simulink model "ZEH_PV_grid"  (R2020a)
settings: Solver=VariableStepAuto  StartTime=0.0  StopTime=24*60*60  RelTol=1e-3
InitFcn:
  | SENSE2_dat
values from neighbouring files (symbols this model uses):
  apv = [72 76 288 252 0 0 40 360 460 168 84]  *1E2    [ZEH_dat_summer.m]    (also in ZEH_dat_winter.m)
  cab = [0.206 0.29 0.36 285 335 ... (first row only)    [ZEH_dat_summer.m]    (also in ZEH_dat_winter.m)
  cons = [0.64,0.60,0.58,0.56,0.56,0.58,0.64,0.76,0.87,0.95,0.99,1.00,0.99,1.00,1.00,0.97,0.96,0.96,0.93,0.92,0.92,0.93,0.87,0.72]    [ZEH_dat_summer.m]    (also in ZEH_dat_winter.m = [0.67,0.63,0.60,0.59,0.59,0.60,0.74,0.86,0.85,0.96,0.96,0.95)
  inic = 0.00095    [ZEH_dat_summer.m]    (also in ZEH_dat_winter.m)
  irr = [0,0,0,0,0,0,0,0,0,0,0,0,0,0,0,0,0,0,0,0,0,0,0,0,0,0,0,0,0,0,0,0,0,0,0,0,0,0,0,0,0,0,0,0,0,0,0,0,0,0,0,0,0,0,0,0,0,0,0,0,0,0,0,0,0,0,0,0,0,0,0,0,0,0,0,0,0,0,0,0,0,0,0,0,0,0,0,0,0,0,0,0,0,0,0,0,0,0,0,0,0,0,0,0,0,0,0,0,0,0,0,0,0,0,0,0,0,0,0,0,0,0,0,0,0,0,0,0,0,0,0,0,0,0,0,0,0,0,0,0,0,0,0,0,0,0,0,0,0,0,0,0,0,0,0,0,0,0,0,0,0,0,0,0,0,0,0,0,0,0,0,0,0,0,0,0,0,0,0,0,0,0,0,0,0,0,0,0,0,0,0,0,0,0,0,0,0,0,0,0 ...(+12851 chars)    [ZEH_dat_summer.m]    (also in ZEH_dat_winter.m = zeros(1,length(irr)))
  lp = 0.002    [ZEH_dat_summer.m]    (also in ZEH_dat_winter.m)
  SL = [7.57 8.06 30.73 53.01 133.26 219.22 4.00 37.53 48.38 17.80 9.04]*1E-3    [ZEH_dat_summer.m]    (also in ZEH_dat_winter.m)
  time = [1,1.01666666666667,1.03333333333333,1.05000000000000,1.06666666666667,1.08333333333333,1.10000000000000,1.11666666666667,1.13333333333333,1.15000000000000,1.16666666666667,1.18333333333333,1.20000000000000,1.21666666666667,1.23333333333333,1.25000000000000,1.26666666666667,1.28333333333333,1.30000000000000,1.31666666666667,1.33333333333333,1.35000000000000,1.36666666666667,1.38333333333333,1.4000 ...(+22733 chars)    [ZEH_dat_summer.m]    (also in ZEH_dat_winter.m)
  to = 0.1    [ZEH_dat_summer.m]    (also in ZEH_dat_winter.m)
undefined symbols (not defined in the file or in its folder): A, B, C, D1, Dd, Delta, j
libraries: powerlib x166, simulink_extras x12, powerlib_meascontrol x11, simulink x2, factslib x2
(part 4 of 5)

== system ZEH_PV_grid/L5/Avoid division by zero ==
  I : Inport
  Complex to Magnitude-Angle : ComplexToMagnitudeAngle
  Magnitude-Angle to Complex : MagnitudeAngleToComplex
  Saturation1 : Saturate  UpperLimit=inf  LowerLimit=1e-6
  O : Outport  VectorParamsAs1DForOutWhenUnconnected=off
  wires:
  I/1 -> Complex to Magnitude-Angle/1
  Saturation1/1 -> Magnitude-Angle to Complex/1
  Complex to Magnitude-Angle/1 -> Saturation1/1
  Magnitude-Angle to Complex/1 -> O/1
  Complex to Magnitude-Angle/2 -> Magnitude-Angle to Complex/2

== system ZEH_PV_grid/L5/Break Alg. Loop 1 ==
  In : Inport
  Complex to Real-Imag : ComplexToRealImag
  Real-Imag to Complex : RealImagToComplex
  imag : Subsystem  mask(Transfer Function with Initial Outputs){N=[1], D=[to  1], Y0=0, U0=0}
      mask prompts: N "Numerator:"; D "Denominator:"; Y0 "Initial output:"; U0 "Initial input:"
      mask help: Vector expressions for numerator, and denominator. Coefficients are in descending powers of s.
      mask init:
      | [A,B,C,Dd]=tf2ss(N,D);if (isempty(Y0));[m,n]=size(A);X0=zeros(1,m); end; if (isempty(U0));[m,p]=size(B);U0=zeros(1,p);end;X0=getxo(A,B,C,Dd,U0,Y0,0);
      mask Help: Specify the initial output for the transfer function.  An optimization routine attempts to determine the appropriate initial states so that the specified initial output is achieved.  For more details, see the m-file getxo.m
      mask Display: dpoly(N,D,'s')
  real : Subsystem  mask(Transfer Function with Initial Outputs){N=[1], D=[to 1], Y0=0, U0=0}
      mask prompts: N "Numerator:"; D "Denominator:"; Y0 "Initial output:"; U0 "Initial input:"
      mask help: Vector expressions for numerator, and denominator. Coefficients are in descending powers of s.
      mask init:
      | [A,B,C,Dd]=tf2ss(N,D);if (isempty(Y0));[m,n]=size(A);X0=zeros(1,m); end; if (isempty(U0));[m,p]=size(B);U0=zeros(1,p);end;X0=getxo(A,B,C,Dd,U0,Y0,0);
      mask Help: Specify the initial output for the transfer function.  An optimization routine attempts to determine the appropriate initial states so that the specified initial output is achieved.  For more details, see the m-file getxo.m
      mask Display: dpoly(N,D,'s')
  Out : Outport  VectorParamsAs1DForOutWhenUnconnected=off
  wires:
  Complex to Real-Imag/1 -> real/1(In1)
  Complex to Real-Imag/2 -> imag/1(In1)
  In/1 -> Complex to Real-Imag/1
  Real-Imag to Complex/1 -> Out/1
  real/1(Out1) -> Real-Imag to Complex/1
  imag/1(Out1) -> Real-Imag to Complex/2

== system ZEH_PV_grid/L5/Load ==
  1 : Constant
  Add : Sum
  Clock : Clock
  Constant : Constant
  Constant1 : Constant  Value=15/24
  Divide : Product  Inputs=*/
  Manual Switch : ManualSwitch
  Mux : Mux  Inputs=2
  P nom : Constant  Value=-nomPower*1e6
  Power consumption : Lookup_n-D  NumberOfTableDimensions=1  BreakpointsForDimension1=[1:timestep/60:24]  BeginIndexSearchUsingPreviousIndexResult=on  Table=datas  InternalRulePriority=Speed  RndMeth=Simplest  InputSameDT=on
  Power factor : Constant  Value=PF^2
  Product : Product
  Product1 : Product
  Scope : Scope
  Second-->Hour : Gain  Gain=1/(60*60)
  Sqrt : Sqrt  SaturateOnIntegerOverflow=on
  Sum : Sum  Inputs=-+
  PQ : Outport  VectorParamsAs1DForOutWhenUnconnected=off
  wires:
  Constant/1 -> Add/2
  1/1 -> Sum/1, Divide/1
  Second-->Hour/1 -> Add/1
  Sum/1 -> Sqrt/1
  Power factor/1 -> Divide/2
  Add/1 -> Power consumption/1
  P nom/1 -> Product/2
  Clock/1 -> Second-->Hour/1
  Sqrt/1 -> Product1/2
  Product/1 -> Product1/1, Mux/1
  Divide/1 -> Sum/2
  Product1/1 -> Mux/2
  Power consumption/1 -> Manual Switch/1
  Manual Switch/1 -> Product/1
  Constant1/1 -> Manual Switch/2
  Mux/1 -> Scope/1, PQ/1

== system ZEH_PV_grid/L6/Avoid division by zero ==
  I : Inport
  Complex to Magnitude-Angle : ComplexToMagnitudeAngle
  Magnitude-Angle to Complex : MagnitudeAngleToComplex
  Saturation1 : Saturate  UpperLimit=inf  LowerLimit=1e-6
  O : Outport  VectorParamsAs1DForOutWhenUnconnected=off
  wires:
  Complex to Magnitude-Angle/2 -> Magnitude-Angle to Complex/2
  Magnitude-Angle to Complex/1 -> O/1
  Complex to Magnitude-Angle/1 -> Saturation1/1
  Saturation1/1 -> Magnitude-Angle to Complex/1
  I/1 -> Complex to Magnitude-Angle/1

== system ZEH_PV_grid/L6/Break Alg. Loop 1 ==
  In : Inport
  Complex to Real-Imag : ComplexToRealImag
  Real-Imag to Complex : RealImagToComplex
  imag : Subsystem  mask(Transfer Function with Initial Outputs){N=[1], D=[to  1], Y0=0, U0=0}
      mask prompts: N "Numerator:"; D "Denominator:"; Y0 "Initial output:"; U0 "Initial input:"
      mask help: Vector expressions for numerator, and denominator. Coefficients are in descending powers of s.
      mask init:
      | [A,B,C,Dd]=tf2ss(N,D);if (isempty(Y0));[m,n]=size(A);X0=zeros(1,m); end; if (isempty(U0));[m,p]=size(B);U0=zeros(1,p);end;X0=getxo(A,B,C,Dd,U0,Y0,0);
      mask Help: Specify the initial output for the transfer function.  An optimization routine attempts to determine the appropriate initial states so that the specified initial output is achieved.  For more details, see the m-file getxo.m
      mask Display: dpoly(N,D,'s')
  real : Subsystem  mask(Transfer Function with Initial Outputs){N=[1], D=[to 1], Y0=0, U0=0}
      mask prompts: N "Numerator:"; D "Denominator:"; Y0 "Initial output:"; U0 "Initial input:"
      mask help: Vector expressions for numerator, and denominator. Coefficients are in descending powers of s.
      mask init:
      | [A,B,C,Dd]=tf2ss(N,D);if (isempty(Y0));[m,n]=size(A);X0=zeros(1,m); end; if (isempty(U0));[m,p]=size(B);U0=zeros(1,p);end;X0=getxo(A,B,C,Dd,U0,Y0,0);
      mask Help: Specify the initial output for the transfer function.  An optimization routine attempts to determine the appropriate initial states so that the specified initial output is achieved.  For more details, see the m-file getxo.m
      mask Display: dpoly(N,D,'s')
  Out : Outport  VectorParamsAs1DForOutWhenUnconnected=off
  wires:
  imag/1(Out1) -> Real-Imag to Complex/2
  real/1(Out1) -> Real-Imag to Complex/1
  Real-Imag to Complex/1 -> Out/1
  In/1 -> Complex to Real-Imag/1
  Complex to Real-Imag/2 -> imag/1(In1)
  Complex to Real-Imag/1 -> real/1(In1)

== system ZEH_PV_grid/L6/Load ==
  1 : Constant
  Add : Sum
  Clock : Clock
  Constant : Constant
  Constant1 : Constant  Value=15/24
  Divide : Product  Inputs=*/
  Manual Switch : ManualSwitch
  Mux : Mux  Inputs=2
  P nom : Constant  Value=-nomPower*1e6
  Power consumption : Lookup_n-D  NumberOfTableDimensions=1  BreakpointsForDimension1=[1:timestep/60:24]  BeginIndexSearchUsingPreviousIndexResult=on  Table=datas  InternalRulePriority=Speed  RndMeth=Simplest  InputSameDT=on
  Power factor : Constant  Value=PF^2
  Product : Product
  Product1 : Product
  Scope : Scope
  Second-->Hour : Gain  Gain=1/(60*60)
  Sqrt : Sqrt  SaturateOnIntegerOverflow=on
  Sum : Sum  Inputs=-+
  PQ : Outport  VectorParamsAs1DForOutWhenUnconnected=off
  wires:
  Mux/1 -> PQ/1, Scope/1
  Constant1/1 -> Manual Switch/2
  Manual Switch/1 -> Product/1
  Power consumption/1 -> Manual Switch/1
  Product1/1 -> Mux/2
  Divide/1 -> Sum/2
  Product/1 -> Mux/1, Product1/1
  Sqrt/1 -> Product1/2
  Clock/1 -> Second-->Hour/1
  P nom/1 -> Product/2
  Add/1 -> Power consumption/1
  Power factor/1 -> Divide/2
  Sum/1 -> Sqrt/1
  Second-->Hour/1 -> Add/1
  1/1 -> Divide/1, Sum/1
  Constant/1 -> Add/2

== system ZEH_PV_grid/L7/Avoid division by zero ==
  I : Inport
  Complex to Magnitude-Angle : ComplexToMagnitudeAngle
  Magnitude-Angle to Complex : MagnitudeAngleToComplex
  Saturation1 : Saturate  UpperLimit=inf  LowerLimit=1e-6
  O : Outport  VectorParamsAs1DForOutWhenUnconnected=off
  wires:
  I/1 -> Complex to Magnitude-Angle/1
  Saturation1/1 -> Magnitude-Angle to Complex/1
  Complex to Magnitude-Angle/1 -> Saturation1/1
  Magnitude-Angle to Complex/1 -> O/1
  Complex to Magnitude-Angle/2 -> Magnitude-Angle to Complex/2

== system ZEH_PV_grid/L7/Break Alg. Loop 1 ==
  In : Inport
  Complex to Real-Imag : ComplexToRealImag
  Real-Imag to Complex : RealImagToComplex
  imag : Subsystem  mask(Transfer Function with Initial Outputs){N=[1], D=[to  1], Y0=0, U0=0}
      mask prompts: N "Numerator:"; D "Denominator:"; Y0 "Initial output:"; U0 "Initial input:"
      mask help: Vector expressions for numerator, and denominator. Coefficients are in descending powers of s.
      mask init:
      | [A,B,C,Dd]=tf2ss(N,D);if (isempty(Y0));[m,n]=size(A);X0=zeros(1,m); end; if (isempty(U0));[m,p]=size(B);U0=zeros(1,p);end;X0=getxo(A,B,C,Dd,U0,Y0,0);
      mask Help: Specify the initial output for the transfer function.  An optimization routine attempts to determine the appropriate initial states so that the specified initial output is achieved.  For more details, see the m-file getxo.m
      mask Display: dpoly(N,D,'s')
  real : Subsystem  mask(Transfer Function with Initial Outputs){N=[1], D=[to 1], Y0=0, U0=0}
      mask prompts: N "Numerator:"; D "Denominator:"; Y0 "Initial output:"; U0 "Initial input:"
      mask help: Vector expressions for numerator, and denominator. Coefficients are in descending powers of s.
      mask init:
      | [A,B,C,Dd]=tf2ss(N,D);if (isempty(Y0));[m,n]=size(A);X0=zeros(1,m); end; if (isempty(U0));[m,p]=size(B);U0=zeros(1,p);end;X0=getxo(A,B,C,Dd,U0,Y0,0);
      mask Help: Specify the initial output for the transfer function.  An optimization routine attempts to determine the appropriate initial states so that the specified initial output is achieved.  For more details, see the m-file getxo.m
      mask Display: dpoly(N,D,'s')
  Out : Outport  VectorParamsAs1DForOutWhenUnconnected=off
  wires:
  Complex to Real-Imag/1 -> real/1(In1)
  Complex to Real-Imag/2 -> imag/1(In1)
  In/1 -> Complex to Real-Imag/1
  Real-Imag to Complex/1 -> Out/1
  real/1(Out1) -> Real-Imag to Complex/1
  imag/1(Out1) -> Real-Imag to Complex/2

== system ZEH_PV_grid/L7/Load ==
  1 : Constant
  Add : Sum
  Clock : Clock
  Constant : Constant
  Constant1 : Constant  Value=15/24
  Divide : Product  Inputs=*/
  Manual Switch : ManualSwitch
  Mux : Mux  Inputs=2
  P nom : Constant  Value=-nomPower*1e6
  Power consumption : Lookup_n-D  NumberOfTableDimensions=1  BreakpointsForDimension1=[1:timestep/60:24]  BeginIndexSearchUsingPreviousIndexResult=on  Table=datas  InternalRulePriority=Speed  RndMeth=Simplest  InputSameDT=on
  Power factor : Constant  Value=PF^2
  Product : Product
  Product1 : Product
  Scope : Scope
  Second-->Hour : Gain  Gain=1/(60*60)
  Sqrt : Sqrt  SaturateOnIntegerOverflow=on
  Sum : Sum  Inputs=-+
  PQ : Outport  VectorParamsAs1DForOutWhenUnconnected=off
  wires:
  Constant/1 -> Add/2
  1/1 -> Sum/1, Divide/1
  Second-->Hour/1 -> Add/1
  Sum/1 -> Sqrt/1
  Power factor/1 -> Divide/2
  Add/1 -> Power consumption/1
  P nom/1 -> Product/2
  Clock/1 -> Second-->Hour/1
  Sqrt/1 -> Product1/2
  Product/1 -> Product1/1, Mux/1
  Divide/1 -> Sum/2
  Product1/1 -> Mux/2
  Power consumption/1 -> Manual Switch/1
  Manual Switch/1 -> Product/1
  Constant1/1 -> Manual Switch/2
  Mux/1 -> Scope/1, PQ/1

== system ZEH_PV_grid/L8/Avoid division by zero ==
  I : Inport
  Complex to Magnitude-Angle : ComplexToMagnitudeAngle
  Magnitude-Angle to Complex : MagnitudeAngleToComplex
  Saturation1 : Saturate  UpperLimit=inf  LowerLimit=1e-6
  O : Outport  VectorParamsAs1DForOutWhenUnconnected=off
  wires:
  Complex to Magnitude-Angle/2 -> Magnitude-Angle to Complex/2
  Magnitude-Angle to Complex/1 -> O/1
  Complex to Magnitude-Angle/1 -> Saturation1/1
  Saturation1/1 -> Magnitude-Angle to Complex/1
  I/1 -> Complex to Magnitude-Angle/1

== system ZEH_PV_grid/L8/Break Alg. Loop 1 ==
  In : Inport
  Complex to Real-Imag : ComplexToRealImag
  Real-Imag to Complex : RealImagToComplex
  imag : Subsystem  mask(Transfer Function with Initial Outputs){N=[1], D=[to  1], Y0=0, U0=0}
      mask prompts: N "Numerator:"; D "Denominator:"; Y0 "Initial output:"; U0 "Initial input:"
      mask help: Vector expressions for numerator, and denominator. Coefficients are in descending powers of s.
      mask init:
      | [A,B,C,Dd]=tf2ss(N,D);if (isempty(Y0));[m,n]=size(A);X0=zeros(1,m); end; if (isempty(U0));[m,p]=size(B);U0=zeros(1,p);end;X0=getxo(A,B,C,Dd,U0,Y0,0);
      mask Help: Specify the initial output for the transfer function.  An optimization routine attempts to determine the appropriate initial states so that the specified initial output is achieved.  For more details, see the m-file getxo.m
      mask Display: dpoly(N,D,'s')
  real : Subsystem  mask(Transfer Function with Initial Outputs){N=[1], D=[to 1], Y0=0, U0=0}
      mask prompts: N "Numerator:"; D "Denominator:"; Y0 "Initial output:"; U0 "Initial input:"
      mask help: Vector expressions for numerator, and denominator. Coefficients are in descending powers of s.
      mask init:
      | [A,B,C,Dd]=tf2ss(N,D);if (isempty(Y0));[m,n]=size(A);X0=zeros(1,m); end; if (isempty(U0));[m,p]=size(B);U0=zeros(1,p);end;X0=getxo(A,B,C,Dd,U0,Y0,0);
      mask Help: Specify the initial output for the transfer function.  An optimization routine attempts to determine the appropriate initial states so that the specified initial output is achieved.  For more details, see the m-file getxo.m
      mask Display: dpoly(N,D,'s')
  Out : Outport  VectorParamsAs1DForOutWhenUnconnected=off
  wires:
  imag/1(Out1) -> Real-Imag to Complex/2
  real/1(Out1) -> Real-Imag to Complex/1
  Real-Imag to Complex/1 -> Out/1
  In/1 -> Complex to Real-Imag/1
  Complex to Real-Imag/2 -> imag/1(In1)
  Complex to Real-Imag/1 -> real/1(In1)

== system ZEH_PV_grid/L8/Load ==
  1 : Constant
  Add : Sum
  Clock : Clock
  Constant : Constant
  Constant1 : Constant  Value=15/24
  Divide : Product  Inputs=*/
  Manual Switch : ManualSwitch
  Mux : Mux  Inputs=2
  P nom : Constant  Value=-nomPower*1e6
  Power consumption : Lookup_n-D  NumberOfTableDimensions=1  BreakpointsForDimension1=[1:timestep/60:24]  BeginIndexSearchUsingPreviousIndexResult=on  Table=datas  InternalRulePriority=Speed  RndMeth=Simplest  InputSameDT=on
  Power factor : Constant  Value=PF^2
  Product : Product
  Product1 : Product
  Scope : Scope
  Second-->Hour : Gain  Gain=1/(60*60)
  Sqrt : Sqrt  SaturateOnIntegerOverflow=on
  Sum : Sum  Inputs=-+
  PQ : Outport  VectorParamsAs1DForOutWhenUnconnected=off
  wires:
  Mux/1 -> PQ/1, Scope/1
  Constant1/1 -> Manual Switch/2
  Manual Switch/1 -> Product/1
  Power consumption/1 -> Manual Switch/1
  Product1/1 -> Mux/2
  Divide/1 -> Sum/2
  Product/1 -> Mux/1, Product1/1
  Sqrt/1 -> Product1/2
  Clock/1 -> Second-->Hour/1
  P nom/1 -> Product/2
  Add/1 -> Power consumption/1
  Power factor/1 -> Divide/2
  Sum/1 -> Sqrt/1
  Second-->Hour/1 -> Add/1
  1/1 -> Divide/1, Sum/1
  Constant/1 -> Add/2

== system ZEH_PV_grid/L9/Avoid division by zero ==
  I : Inport
  Complex to Magnitude-Angle : ComplexToMagnitudeAngle
  Magnitude-Angle to Complex : MagnitudeAngleToComplex
  Saturation1 : Saturate  UpperLimit=inf  LowerLimit=1e-6
  O : Outport  VectorParamsAs1DForOutWhenUnconnected=off
  wires:
  I/1 -> Complex to Magnitude-Angle/1
  Saturation1/1 -> Magnitude-Angle to Complex/1
  Complex to Magnitude-Angle/1 -> Saturation1/1
  Magnitude-Angle to Complex/1 -> O/1
  Complex to Magnitude-Angle/2 -> Magnitude-Angle to Complex/2

== system ZEH_PV_grid/L9/Break Alg. Loop 1 ==
  In : Inport
  Complex to Real-Imag : ComplexToRealImag
  Real-Imag to Complex : RealImagToComplex
  imag : Subsystem  mask(Transfer Function with Initial Outputs){N=[1], D=[to  1], Y0=0, U0=0}
      mask prompts: N "Numerator:"; D "Denominator:"; Y0 "Initial output:"; U0 "Initial input:"
      mask help: Vector expressions for numerator, and denominator. Coefficients are in descending powers of s.
      mask init:
      | [A,B,C,Dd]=tf2ss(N,D);if (isempty(Y0));[m,n]=size(A);X0=zeros(1,m); end; if (isempty(U0));[m,p]=size(B);U0=zeros(1,p);end;X0=getxo(A,B,C,Dd,U0,Y0,0);
      mask Help: Specify the initial output for the transfer function.  An optimization routine attempts to determine the appropriate initial states so that the specified initial output is achieved.  For more details, see the m-file getxo.m
      mask Display: dpoly(N,D,'s')
  real : Subsystem  mask(Transfer Function with Initial Outputs){N=[1], D=[to 1], Y0=0, U0=0}
      mask prompts: N "Numerator:"; D "Denominator:"; Y0 "Initial output:"; U0 "Initial input:"
      mask help: Vector expressions for numerator, and denominator. Coefficients are in descending powers of s.
      mask init:
      | [A,B,C,Dd]=tf2ss(N,D);if (isempty(Y0));[m,n]=size(A);X0=zeros(1,m); end; if (isempty(U0));[m,p]=size(B);U0=zeros(1,p);end;X0=getxo(A,B,C,Dd,U0,Y0,0);
      mask Help: Specify the initial output for the transfer function.  An optimization routine attempts to determine the appropriate initial states so that the specified initial output is achieved.  For more details, see the m-file getxo.m
      mask Display: dpoly(N,D,'s')
  Out : Outport  VectorParamsAs1DForOutWhenUnconnected=off
  wires:
  Complex to Real-Imag/1 -> real/1(In1)
  Complex to Real-Imag/2 -> imag/1(In1)
  In/1 -> Complex to Real-Imag/1
  Real-Imag to Complex/1 -> Out/1
  real/1(Out1) -> Real-Imag to Complex/1
  imag/1(Out1) -> Real-Imag to Complex/2

== system ZEH_PV_grid/L9/Load ==
  1 : Constant
  Add : Sum
  Clock : Clock
  Constant : Constant
  Constant1 : Constant  Value=15/24
  Divide : Product  Inputs=*/
  Manual Switch : ManualSwitch
  Mux : Mux  Inputs=2
  P nom : Constant  Value=-nomPower*1e6
  Power consumption : Lookup_n-D  NumberOfTableDimensions=1  BreakpointsForDimension1=[1:timestep/60:24]  BeginIndexSearchUsingPreviousIndexResult=on  Table=datas  InternalRulePriority=Speed  RndMeth=Simplest  InputSameDT=on
  Power factor : Constant  Value=PF^2
  Product : Product
  Product1 : Product
  Scope : Scope
  Second-->Hour : Gain  Gain=1/(60*60)
  Sqrt : Sqrt  SaturateOnIntegerOverflow=on
  Sum : Sum  Inputs=-+
  PQ : Outport  VectorParamsAs1DForOutWhenUnconnected=off
  wires:
  Constant/1 -> Add/2
  1/1 -> Sum/1, Divide/1
  Second-->Hour/1 -> Add/1
  Sum/1 -> Sqrt/1
  Power factor/1 -> Divide/2
  Add/1 -> Power consumption/1
  P nom/1 -> Product/2
  Clock/1 -> Second-->Hour/1
  Sqrt/1 -> Product1/2
  Product/1 -> Product1/1, Mux/1
  Divide/1 -> Sum/2
  Product1/1 -> Mux/2
  Power consumption/1 -> Manual Switch/1
  Manual Switch/1 -> Product/1
  Constant1/1 -> Manual Switch/2
  Mux/1 -> Scope/1, PQ/1

== system ZEH_PV_grid/PV1/Avoid division by zero ==
  I : Inport
  Complex to Magnitude-Angle : ComplexToMagnitudeAngle
  Magnitude-Angle to Complex : MagnitudeAngleToComplex
  Saturation1 : Saturate  UpperLimit=inf  LowerLimit=1e-6
  O : Outport  VectorParamsAs1DForOutWhenUnconnected=off
  wires:
  Complex to Magnitude-Angle/2 -> Magnitude-Angle to Complex/2
  Magnitude-Angle to Complex/1 -> O/1
  Complex to Magnitude-Angle/1 -> Saturation1/1
  Saturation1/1 -> Magnitude-Angle to Complex/1
  I/1 -> Complex to Magnitude-Angle/1

== system ZEH_PV_grid/PV1/Break Alg. Loop 1 ==
  In : Inport
  Complex to Real-Imag : ComplexToRealImag
  Real-Imag to Complex : RealImagToComplex
  imag : Subsystem  mask(Transfer Function with Initial Outputs){N=[1], D=[to  1], Y0=0, U0=0}
      mask prompts: N "Numerator:"; D "Denominator:"; Y0 "Initial output:"; U0 "Initial input:"
      mask help: Vector expressions for numerator, and denominator. Coefficients are in descending powers of s.
      mask init:
      | [A,B,C,Dd]=tf2ss(N,D);if (isempty(Y0));[m,n]=size(A);X0=zeros(1,m); end; if (isempty(U0));[m,p]=size(B);U0=zeros(1,p);end;X0=getxo(A,B,C,Dd,U0,Y0,0);
      mask Help: Specify the initial output for the transfer function.  An optimization routine attempts to determine the appropriate initial states so that the specified initial output is achieved.  For more details, see the m-file getxo.m
      mask Display: dpoly(N,D,'s')
  real : Subsystem  mask(Transfer Function with Initial Outputs){N=[1], D=[to 1], Y0=0, U0=0}
      mask prompts: N "Numerator:"; D "Denominator:"; Y0 "Initial output:"; U0 "Initial input:"
      mask help: Vector expressions for numerator, and denominator. Coefficients are in descending powers of s.
      mask init:
      | [A,B,C,Dd]=tf2ss(N,D);if (isempty(Y0));[m,n]=size(A);X0=zeros(1,m); end; if (isempty(U0));[m,p]=size(B);U0=zeros(1,p);end;X0=getxo(A,B,C,Dd,U0,Y0,0);
      mask Help: Specify the initial output for the transfer function.  An optimization routine attempts to determine the appropriate initial states so that the specified initial output is achieved.  For more details, see the m-file getxo.m
      mask Display: dpoly(N,D,'s')
  Out : Outport  VectorParamsAs1DForOutWhenUnconnected=off
  wires:
  Complex to Real-Imag/1 -> real/1(In1)
  Complex to Real-Imag/2 -> imag/1(In1)
  In/1 -> Complex to Real-Imag/1
  Real-Imag to Complex/1 -> Out/1
  real/1(Out1) -> Real-Imag to Complex/1
  imag/1(Out1) -> Real-Imag to Complex/2

== system ZEH_PV_grid/PV10/Avoid division by zero ==
  I : Inport
  Complex to Magnitude-Angle : ComplexToMagnitudeAngle
  Magnitude-Angle to Complex : MagnitudeAngleToComplex
  Saturation1 : Saturate  UpperLimit=inf  LowerLimit=1e-6
  O : Outport  VectorParamsAs1DForOutWhenUnconnected=off
  wires:
  I/1 -> Complex to Magnitude-Angle/1
  Saturation1/1 -> Magnitude-Angle to Complex/1
  Complex to Magnitude-Angle/1 -> Saturation1/1
  Magnitude-Angle to Complex/1 -> O/1
  Complex to Magnitude-Angle/2 -> Magnitude-Angle to Complex/2

== system ZEH_PV_grid/PV10/Break Alg. Loop 1 ==
  In : Inport
  Complex to Real-Imag : ComplexToRealImag
  Real-Imag to Complex : RealImagToComplex
  imag : Subsystem  mask(Transfer Function with Initial Outputs){N=[1], D=[to  1], Y0=0, U0=0}
      mask prompts: N "Numerator:"; D "Denominator:"; Y0 "Initial output:"; U0 "Initial input:"
      mask help: Vector expressions for numerator, and denominator. Coefficients are in descending powers of s.
      mask init:
      | [A,B,C,Dd]=tf2ss(N,D);if (isempty(Y0));[m,n]=size(A);X0=zeros(1,m); end; if (isempty(U0));[m,p]=size(B);U0=zeros(1,p);end;X0=getxo(A,B,C,Dd,U0,Y0,0);
      mask Help: Specify the initial output for the transfer function.  An optimization routine attempts to determine the appropriate initial states so that the specified initial output is achieved.  For more details, see the m-file getxo.m
      mask Display: dpoly(N,D,'s')
  real : Subsystem  mask(Transfer Function with Initial Outputs){N=[1], D=[to 1], Y0=0, U0=0}
      mask prompts: N "Numerator:"; D "Denominator:"; Y0 "Initial output:"; U0 "Initial input:"
      mask help: Vector expressions for numerator, and denominator. Coefficients are in descending powers of s.
      mask init:
      | [A,B,C,Dd]=tf2ss(N,D);if (isempty(Y0));[m,n]=size(A);X0=zeros(1,m); end; if (isempty(U0));[m,p]=size(B);U0=zeros(1,p);end;X0=getxo(A,B,C,Dd,U0,Y0,0);
      mask Help: Specify the initial output for the transfer function.  An optimization routine attempts to determine the appropriate initial states so that the specified initial output is achieved.  For more details, see the m-file getxo.m
      mask Display: dpoly(N,D,'s')
  Out : Outport  VectorParamsAs1DForOutWhenUnconnected=off
  wires:
  imag/1(Out1) -> Real-Imag to Complex/2
  real/1(Out1) -> Real-Imag to Complex/1
  Real-Imag to Complex/1 -> Out/1
  In/1 -> Complex to Real-Imag/1
  Complex to Real-Imag/2 -> imag/1(In1)
  Complex to Real-Imag/1 -> real/1(In1)

== system ZEH_PV_grid/PV11/Avoid division by zero ==
  I : Inport
  Complex to Magnitude-Angle : ComplexToMagnitudeAngle
  Magnitude-Angle to Complex : MagnitudeAngleToComplex
  Saturation1 : Saturate  UpperLimit=inf  LowerLimit=1e-6
  O : Outport  VectorParamsAs1DForOutWhenUnconnected=off
  wires:
  Complex to Magnitude-Angle/2 -> Magnitude-Angle to Complex/2
  Magnitude-Angle to Complex/1 -> O/1
  Complex to Magnitude-Angle/1 -> Saturation1/1
  Saturation1/1 -> Magnitude-Angle to Complex/1
  I/1 -> Complex to Magnitude-Angle/1

== system ZEH_PV_grid/PV11/Break Alg. Loop 1 ==
  In : Inport
  Complex to Real-Imag : ComplexToRealImag
  Real-Imag to Complex : RealImagToComplex
  imag : Subsystem  mask(Transfer Function with Initial Outputs){N=[1], D=[to  1], Y0=0, U0=0}
      mask prompts: N "Numerator:"; D "Denominator:"; Y0 "Initial output:"; U0 "Initial input:"
      mask help: Vector expressions for numerator, and denominator. Coefficients are in descending powers of s.
      mask init:
      | [A,B,C,Dd]=tf2ss(N,D);if (isempty(Y0));[m,n]=size(A);X0=zeros(1,m); end; if (isempty(U0));[m,p]=size(B);U0=zeros(1,p);end;X0=getxo(A,B,C,Dd,U0,Y0,0);
      mask Help: Specify the initial output for the transfer function.  An optimization routine attempts to determine the appropriate initial states so that the specified initial output is achieved.  For more details, see the m-file getxo.m
      mask Display: dpoly(N,D,'s')
  real : Subsystem  mask(Transfer Function with Initial Outputs){N=[1], D=[to 1], Y0=0, U0=0}
      mask prompts: N "Numerator:"; D "Denominator:"; Y0 "Initial output:"; U0 "Initial input:"
      mask help: Vector expressions for numerator, and denominator. Coefficients are in descending powers of s.
      mask init:
      | [A,B,C,Dd]=tf2ss(N,D);if (isempty(Y0));[m,n]=size(A);X0=zeros(1,m); end; if (isempty(U0));[m,p]=size(B);U0=zeros(1,p);end;X0=getxo(A,B,C,Dd,U0,Y0,0);
      mask Help: Specify the initial output for the transfer function.  An optimization routine attempts to determine the appropriate initial states so that the specified initial output is achieved.  For more details, see the m-file getxo.m
      mask Display: dpoly(N,D,'s')
  Out : Outport  VectorParamsAs1DForOutWhenUnconnected=off
  wires:
  Complex to Real-Imag/1 -> real/1(In1)
  Complex to Real-Imag/2 -> imag/1(In1)
  In/1 -> Complex to Real-Imag/1
  Real-Imag to Complex/1 -> Out/1
  real/1(Out1) -> Real-Imag to Complex/1
  imag/1(Out1) -> Real-Imag to Complex/2

== system ZEH_PV_grid/PV2/Avoid division by zero ==
  I : Inport
  Complex to Magnitude-Angle : ComplexToMagnitudeAngle
  Magnitude-Angle to Complex : MagnitudeAngleToComplex
  Saturation1 : Saturate  UpperLimit=inf  LowerLimit=1e-6
  O : Outport  VectorParamsAs1DForOutWhenUnconnected=off
  wires:
  I/1 -> Complex to Magnitude-Angle/1
  Saturation1/1 -> Magnitude-Angle to Complex/1
  Complex to Magnitude-Angle/1 -> Saturation1/1
  Magnitude-Angle to Complex/1 -> O/1
  Complex to Magnitude-Angle/2 -> Magnitude-Angle to Complex/2

== system ZEH_PV_grid/PV2/Break Alg. Loop 1 ==
  In : Inport
  Complex to Real-Imag : ComplexToRealImag
  Real-Imag to Complex : RealImagToComplex
  imag : Subsystem  mask(Transfer Function with Initial Outputs){N=[1], D=[to  1], Y0=0, U0=0}
      mask prompts: N "Numerator:"; D "Denominator:"; Y0 "Initial output:"; U0 "Initial input:"
      mask help: Vector expressions for numerator, and denominator. Coefficients are in descending powers of s.
      mask init:
      | [A,B,C,Dd]=tf2ss(N,D);if (isempty(Y0));[m,n]=size(A);X0=zeros(1,m); end; if (isempty(U0));[m,p]=size(B);U0=zeros(1,p);end;X0=getxo(A,B,C,Dd,U0,Y0,0);
      mask Help: Specify the initial output for the transfer function.  An optimization routine attempts to determine the appropriate initial states so that the specified initial output is achieved.  For more details, see the m-file getxo.m
      mask Display: dpoly(N,D,'s')
  real : Subsystem  mask(Transfer Function with Initial Outputs){N=[1], D=[to 1], Y0=0, U0=0}
      mask prompts: N "Numerator:"; D "Denominator:"; Y0 "Initial output:"; U0 "Initial input:"
      mask help: Vector expressions for numerator, and denominator. Coefficients are in descending powers of s.
      mask init:
      | [A,B,C,Dd]=tf2ss(N,D);if (isempty(Y0));[m,n]=size(A);X0=zeros(1,m); end; if (isempty(U0));[m,p]=size(B);U0=zeros(1,p);end;X0=getxo(A,B,C,Dd,U0,Y0,0);
      mask Help: Specify the initial output for the transfer function.  An optimization routine attempts to determine the appropriate initial states so that the specified initial output is achieved.  For more details, see the m-file getxo.m
      mask Display: dpoly(N,D,'s')
  Out : Outport  VectorParamsAs1DForOutWhenUnconnected=off
  wires:
  imag/1(Out1) -> Real-Imag to Complex/2
  real/1(Out1) -> Real-Imag to Complex/1
  Real-Imag to Complex/1 -> Out/1
  In/1 -> Complex to Real-Imag/1
  Complex to Real-Imag/2 -> imag/1(In1)
  Complex to Real-Imag/1 -> real/1(In1)

== system ZEH_PV_grid/PV3/Avoid division by zero ==
  I : Inport
  Complex to Magnitude-Angle : ComplexToMagnitudeAngle
  Magnitude-Angle to Complex : MagnitudeAngleToComplex
  Saturation1 : Saturate  UpperLimit=inf  LowerLimit=1e-6
  O : Outport  VectorParamsAs1DForOutWhenUnconnected=off
  wires:
  Complex to Magnitude-Angle/2 -> Magnitude-Angle to Complex/2
  Magnitude-Angle to Complex/1 -> O/1
  Complex to Magnitude-Angle/1 -> Saturation1/1
  Saturation1/1 -> Magnitude-Angle to Complex/1
  I/1 -> Complex to Magnitude-Angle/1

== system ZEH_PV_grid/PV3/Break Alg. Loop 1 ==
  In : Inport
  Complex to Real-Imag : ComplexToRealImag
  Real-Imag to Complex : RealImagToComplex
  imag : Subsystem  mask(Transfer Function with Initial Outputs){N=[1], D=[to  1], Y0=0, U0=0}
      mask prompts: N "Numerator:"; D "Denominator:"; Y0 "Initial output:"; U0 "Initial input:"
      mask help: Vector expressions for numerator, and denominator. Coefficients are in descending powers of s.
      mask init:
      | [A,B,C,Dd]=tf2ss(N,D);if (isempty(Y0));[m,n]=size(A);X0=zeros(1,m); end; if (isempty(U0));[m,p]=size(B);U0=zeros(1,p);end;X0=getxo(A,B,C,Dd,U0,Y0,0);
      mask Help: Specify the initial output for the transfer function.  An optimization routine attempts to determine the appropriate initial states so that the specified initial output is achieved.  For more details, see the m-file getxo.m
      mask Display: dpoly(N,D,'s')
  real : Subsystem  mask(Transfer Function with Initial Outputs){N=[1], D=[to 1], Y0=0, U0=0}
      mask prompts: N "Numerator:"; D "Denominator:"; Y0 "Initial output:"; U0 "Initial input:"
      mask help: Vector expressions for numerator, and denominator. Coefficients are in descending powers of s.
      mask init:
      | [A,B,C,Dd]=tf2ss(N,D);if (isempty(Y0));[m,n]=size(A);X0=zeros(1,m); end; if (isempty(U0));[m,p]=size(B);U0=zeros(1,p);end;X0=getxo(A,B,C,Dd,U0,Y0,0);
      mask Help: Specify the initial output for the transfer function.  An optimization routine attempts to determine the appropriate initial states so that the specified initial output is achieved.  For more details, see the m-file getxo.m
      mask Display: dpoly(N,D,'s')
  Out : Outport  VectorParamsAs1DForOutWhenUnconnected=off
  wires:
  Complex to Real-Imag/1 -> real/1(In1)
  Complex to Real-Imag/2 -> imag/1(In1)
  In/1 -> Complex to Real-Imag/1
  Real-Imag to Complex/1 -> Out/1
  real/1(Out1) -> Real-Imag to Complex/1
  imag/1(Out1) -> Real-Imag to Complex/2

== system ZEH_PV_grid/PV4/Avoid division by zero ==
  I : Inport
  Complex to Magnitude-Angle : ComplexToMagnitudeAngle
  Magnitude-Angle to Complex : MagnitudeAngleToComplex
  Saturation1 : Saturate  UpperLimit=inf  LowerLimit=1e-6
  O : Outport  VectorParamsAs1DForOutWhenUnconnected=off
  wires:
  I/1 -> Complex to Magnitude-Angle/1
  Saturation1/1 -> Magnitude-Angle to Complex/1
  Complex to Magnitude-Angle/1 -> Saturation1/1
  Magnitude-Angle to Complex/1 -> O/1
  Complex to Magnitude-Angle/2 -> Magnitude-Angle to Complex/2

== system ZEH_PV_grid/PV4/Break Alg. Loop 1 ==
  In : Inport
  Complex to Real-Imag : ComplexToRealImag
  Real-Imag to Complex : RealImagToComplex
  imag : Subsystem  mask(Transfer Function with Initial Outputs){N=[1], D=[to  1], Y0=0, U0=0}
      mask prompts: N "Numerator:"; D "Denominator:"; Y0 "Initial output:"; U0 "Initial input:"
      mask help: Vector expressions for numerator, and denominator. Coefficients are in descending powers of s.
      mask init:
      | [A,B,C,Dd]=tf2ss(N,D);if (isempty(Y0));[m,n]=size(A);X0=zeros(1,m); end; if (isempty(U0));[m,p]=size(B);U0=zeros(1,p);end;X0=getxo(A,B,C,Dd,U0,Y0,0);
      mask Help: Specify the initial output for the transfer function.  An optimization routine attempts to determine the appropriate initial states so that the specified initial output is achieved.  For more details, see the m-file getxo.m
      mask Display: dpoly(N,D,'s')
  real : Subsystem  mask(Transfer Function with Initial Outputs){N=[1], D=[to 1], Y0=0, U0=0}
      mask prompts: N "Numerator:"; D "Denominator:"; Y0 "Initial output:"; U0 "Initial input:"
      mask help: Vector expressions for numerator, and denominator. Coefficients are in descending powers of s.
      mask init:
      | [A,B,C,Dd]=tf2ss(N,D);if (isempty(Y0));[m,n]=size(A);X0=zeros(1,m); end; if (isempty(U0));[m,p]=size(B);U0=zeros(1,p);end;X0=getxo(A,B,C,Dd,U0,Y0,0);
      mask Help: Specify the initial output for the transfer function.  An optimization routine attempts to determine the appropriate initial states so that the specified initial output is achieved.  For more details, see the m-file getxo.m
      mask Display: dpoly(N,D,'s')
  Out : Outport  VectorParamsAs1DForOutWhenUnconnected=off
  wires:
  imag/1(Out1) -> Real-Imag to Complex/2
  real/1(Out1) -> Real-Imag to Complex/1
  Real-Imag to Complex/1 -> Out/1
  In/1 -> Complex to Real-Imag/1
  Complex to Real-Imag/2 -> imag/1(In1)
  Complex to Real-Imag/1 -> real/1(In1)

== system ZEH_PV_grid/PV5/Avoid division by zero ==
  I : Inport
  Complex to Magnitude-Angle : ComplexToMagnitudeAngle
  Magnitude-Angle to Complex : MagnitudeAngleToComplex
  Saturation1 : Saturate  UpperLimit=inf  LowerLimit=1e-6
  O : Outport  VectorParamsAs1DForOutWhenUnconnected=off
  wires:
  Complex to Magnitude-Angle/2 -> Magnitude-Angle to Complex/2
  Magnitude-Angle to Complex/1 -> O/1
  Complex to Magnitude-Angle/1 -> Saturation1/1
  Saturation1/1 -> Magnitude-Angle to Complex/1
  I/1 -> Complex to Magnitude-Angle/1

== system ZEH_PV_grid/PV5/Break Alg. Loop 1 ==
  In : Inport
  Complex to Real-Imag : ComplexToRealImag
  Real-Imag to Complex : RealImagToComplex
  imag : Subsystem  mask(Transfer Function with Initial Outputs){N=[1], D=[to  1], Y0=0, U0=0}
      mask prompts: N "Numerator:"; D "Denominator:"; Y0 "Initial output:"; U0 "Initial input:"
      mask help: Vector expressions for numerator, and denominator. Coefficients are in descending powers of s.
      mask init:
      | [A,B,C,Dd]=tf2ss(N,D);if (isempty(Y0));[m,n]=size(A);X0=zeros(1,m); end; if (isempty(U0));[m,p]=size(B);U0=zeros(1,p);end;X0=getxo(A,B,C,Dd,U0,Y0,0);
      mask Help: Specify the initial output for the transfer function.  An optimization routine attempts to determine the appropriate initial states so that the specified initial output is achieved.  For more details, see the m-file getxo.m
      mask Display: dpoly(N,D,'s')
  real : Subsystem  mask(Transfer Function with Initial Outputs){N=[1], D=[to 1], Y0=0, U0=0}
      mask prompts: N "Numerator:"; D "Denominator:"; Y0 "Initial output:"; U0 "Initial input:"
      mask help: Vector expressions for numerator, and denominator. Coefficients are in descending powers of s.
      mask init:
      | [A,B,C,Dd]=tf2ss(N,D);if (isempty(Y0));[m,n]=size(A);X0=zeros(1,m); end; if (isempty(U0));[m,p]=size(B);U0=zeros(1,p);end;X0=getxo(A,B,C,Dd,U0,Y0,0);
      mask Help: Specify the initial output for the transfer function.  An optimization routine attempts to determine the appropriate initial states so that the specified initial output is achieved.  For more details, see the m-file getxo.m
      mask Display: dpoly(N,D,'s')
  Out : Outport  VectorParamsAs1DForOutWhenUnconnected=off
  wires:
  Complex to Real-Imag/1 -> real/1(In1)
  Complex to Real-Imag/2 -> imag/1(In1)
  In/1 -> Complex to Real-Imag/1
  Real-Imag to Complex/1 -> Out/1
  real/1(Out1) -> Real-Imag to Complex/1
  imag/1(Out1) -> Real-Imag to Complex/2

== system ZEH_PV_grid/PV6/Avoid division by zero ==
  I : Inport
  Complex to Magnitude-Angle : ComplexToMagnitudeAngle
  Magnitude-Angle to Complex : MagnitudeAngleToComplex
  Saturation1 : Saturate  UpperLimit=inf  LowerLimit=1e-6
  O : Outport  VectorParamsAs1DForOutWhenUnconnected=off
  wires:
  I/1 -> Complex to Magnitude-Angle/1
  Saturation1/1 -> Magnitude-Angle to Complex/1
  Complex to Magnitude-Angle/1 -> Saturation1/1
  Magnitude-Angle to Complex/1 -> O/1
  Complex to Magnitude-Angle/2 -> Magnitude-Angle to Complex/2

== system ZEH_PV_grid/PV6/Break Alg. Loop 1 ==
  In : Inport
  Complex to Real-Imag : ComplexToRealImag
  Real-Imag to Complex : RealImagToComplex
  imag : Subsystem  mask(Transfer Function with Initial Outputs){N=[1], D=[to  1], Y0=0, U0=0}
      mask prompts: N "Numerator:"; D "Denominator:"; Y0 "Initial output:"; U0 "Initial input:"
      mask help: Vector expressions for numerator, and denominator. Coefficients are in descending powers of s.
      mask init:
      | [A,B,C,Dd]=tf2ss(N,D);if (isempty(Y0));[m,n]=size(A);X0=zeros(1,m); end; if (isempty(U0));[m,p]=size(B);U0=zeros(1,p);end;X0=getxo(A,B,C,Dd,U0,Y0,0);
      mask Help: Specify the initial output for the transfer function.  An optimization routine attempts to determine the appropriate initial states so that the specified initial output is achieved.  For more details, see the m-file getxo.m
      mask Display: dpoly(N,D,'s')
  real : Subsystem  mask(Transfer Function with Initial Outputs){N=[1], D=[to 1], Y0=0, U0=0}
      mask prompts: N "Numerator:"; D "Denominator:"; Y0 "Initial output:"; U0 "Initial input:"
      mask help: Vector expressions for numerator, and denominator. Coefficients are in descending powers of s.
      mask init:
      | [A,B,C,Dd]=tf2ss(N,D);if (isempty(Y0));[m,n]=size(A);X0=zeros(1,m); end; if (isempty(U0));[m,p]=size(B);U0=zeros(1,p);end;X0=getxo(A,B,C,Dd,U0,Y0,0);
      mask Help: Specify the initial output for the transfer function.  An optimization routine attempts to determine the appropriate initial states so that the specified initial output is achieved.  For more details, see the m-file getxo.m
      mask Display: dpoly(N,D,'s')
  Out : Outport  VectorParamsAs1DForOutWhenUnconnected=off
  wires:
  imag/1(Out1) -> Real-Imag to Complex/2
  real/1(Out1) -> Real-Imag to Complex/1
  Real-Imag to Complex/1 -> Out/1
  In/1 -> Complex to Real-Imag/1
  Complex to Real-Imag/2 -> imag/1(In1)
  Complex to Real-Imag/1 -> real/1(In1)

== system ZEH_PV_grid/PV7/Avoid division by zero ==
  I : Inport
  Complex to Magnitude-Angle : ComplexToMagnitudeAngle
  Magnitude-Angle to Complex : MagnitudeAngleToComplex
  Saturation1 : Saturate  UpperLimit=inf  LowerLimit=1e-6
  O : Outport  VectorParamsAs1DForOutWhenUnconnected=off
  wires:
  Complex to Magnitude-Angle/2 -> Magnitude-Angle to Complex/2
  Magnitude-Angle to Complex/1 -> O/1
  Complex to Magnitude-Angle/1 -> Saturation1/1
  Saturation1/1 -> Magnitude-Angle to Complex/1
  I/1 -> Complex to Magnitude-Angle/1

== system ZEH_PV_grid/PV7/Break Alg. Loop 1 ==
  In : Inport
  Complex to Real-Imag : ComplexToRealImag
  Real-Imag to Complex : RealImagToComplex
  imag : Subsystem  mask(Transfer Function with Initial Outputs){N=[1], D=[to  1], Y0=0, U0=0}
      mask prompts: N "Numerator:"; D "Denominator:"; Y0 "Initial output:"; U0 "Initial input:"
      mask help: Vector expressions for numerator, and denominator. Coefficients are in descending powers of s.
      mask init:
      | [A,B,C,Dd]=tf2ss(N,D);if (isempty(Y0));[m,n]=size(A);X0=zeros(1,m); end; if (isempty(U0));[m,p]=size(B);U0=zeros(1,p);end;X0=getxo(A,B,C,Dd,U0,Y0,0);
      mask Help: Specify the initial output for the transfer function.  An optimization routine attempts to determine the appropriate initial states so that the specified initial output is achieved.  For more details, see the m-file getxo.m
      mask Display: dpoly(N,D,'s')
  real : Subsystem  mask(Transfer Function with Initial Outputs){N=[1], D=[to 1], Y0=0, U0=0}
      mask prompts: N "Numerator:"; D "Denominator:"; Y0 "Initial output:"; U0 "Initial input:"
      mask help: Vector expressions for numerator, and denominator. Coefficients are in descending powers of s.
      mask init:
      | [A,B,C,Dd]=tf2ss(N,D);if (isempty(Y0));[m,n]=size(A);X0=zeros(1,m); end; if (isempty(U0));[m,p]=size(B);U0=zeros(1,p);end;X0=getxo(A,B,C,Dd,U0,Y0,0);
      mask Help: Specify the initial output for the transfer function.  An optimization routine attempts to determine the appropriate initial states so that the specified initial output is achieved.  For more details, see the m-file getxo.m
      mask Display: dpoly(N,D,'s')
  Out : Outport  VectorParamsAs1DForOutWhenUnconnected=off
  wires:
  Complex to Real-Imag/1 -> real/1(In1)
  Complex to Real-Imag/2 -> imag/1(In1)
  In/1 -> Complex to Real-Imag/1
  Real-Imag to Complex/1 -> Out/1
  real/1(Out1) -> Real-Imag to Complex/1
  imag/1(Out1) -> Real-Imag to Complex/2

== system ZEH_PV_grid/PV8/Avoid division by zero ==
  I : Inport
  Complex to Magnitude-Angle : ComplexToMagnitudeAngle
  Magnitude-Angle to Complex : MagnitudeAngleToComplex
  Saturation1 : Saturate  UpperLimit=inf  LowerLimit=1e-6
  O : Outport  VectorParamsAs1DForOutWhenUnconnected=off
  wires:
  I/1 -> Complex to Magnitude-Angle/1
  Saturation1/1 -> Magnitude-Angle to Complex/1
  Complex to Magnitude-Angle/1 -> Saturation1/1
  Magnitude-Angle to Complex/1 -> O/1
  Complex to Magnitude-Angle/2 -> Magnitude-Angle to Complex/2

== system ZEH_PV_grid/PV8/Break Alg. Loop 1 ==
  In : Inport
  Complex to Real-Imag : ComplexToRealImag
  Real-Imag to Complex : RealImagToComplex
  imag : Subsystem  mask(Transfer Function with Initial Outputs){N=[1], D=[to  1], Y0=0, U0=0}
      mask prompts: N "Numerator:"; D "Denominator:"; Y0 "Initial output:"; U0 "Initial input:"
      mask help: Vector expressions for numerator, and denominator. Coefficients are in descending powers of s.
      mask init:
      | [A,B,C,Dd]=tf2ss(N,D);if (isempty(Y0));[m,n]=size(A);X0=zeros(1,m); end; if (isempty(U0));[m,p]=size(B);U0=zeros(1,p);end;X0=getxo(A,B,C,Dd,U0,Y0,0);
      mask Help: Specify the initial output for the transfer function.  An optimization routine attempts to determine the appropriate initial states so that the specified initial output is achieved.  For more details, see the m-file getxo.m
      mask Display: dpoly(N,D,'s')
  real : Subsystem  mask(Transfer Function with Initial Outputs){N=[1], D=[to 1], Y0=0, U0=0}
      mask prompts: N "Numerator:"; D "Denominator:"; Y0 "Initial output:"; U0 "Initial input:"
      mask help: Vector expressions for numerator, and denominator. Coefficients are in descending powers of s.
      mask init:
      | [A,B,C,Dd]=tf2ss(N,D);if (isempty(Y0));[m,n]=size(A);X0=zeros(1,m); end; if (isempty(U0));[m,p]=size(B);U0=zeros(1,p);end;X0=getxo(A,B,C,Dd,U0,Y0,0);
      mask Help: Specify the initial output for the transfer function.  An optimization routine attempts to determine the appropriate initial states so that the specified initial output is achieved.  For more details, see the m-file getxo.m
      mask Display: dpoly(N,D,'s')
  Out : Outport  VectorParamsAs1DForOutWhenUnconnected=off
  wires:
  imag/1(Out1) -> Real-Imag to Complex/2
  real/1(Out1) -> Real-Imag to Complex/1
  Real-Imag to Complex/1 -> Out/1
  In/1 -> Complex to Real-Imag/1
  Complex to Real-Imag/2 -> imag/1(In1)
  Complex to Real-Imag/1 -> real/1(In1)

== system ZEH_PV_grid/PV9/Avoid division by zero ==
  I : Inport
  Complex to Magnitude-Angle : ComplexToMagnitudeAngle
  Magnitude-Angle to Complex : MagnitudeAngleToComplex
  Saturation1 : Saturate  UpperLimit=inf  LowerLimit=1e-6
  O : Outport  VectorParamsAs1DForOutWhenUnconnected=off
  wires:
  Complex to Magnitude-Angle/2 -> Magnitude-Angle to Complex/2
  Magnitude-Angle to Complex/1 -> O/1
  Complex to Magnitude-Angle/1 -> Saturation1/1
  Saturation1/1 -> Magnitude-Angle to Complex/1
  I/1 -> Complex to Magnitude-Angle/1

== system ZEH_PV_grid/PV9/Break Alg. Loop 1 ==
  In : Inport
  Complex to Real-Imag : ComplexToRealImag
  Real-Imag to Complex : RealImagToComplex
  imag : Subsystem  mask(Transfer Function with Initial Outputs){N=[1], D=[to  1], Y0=0, U0=0}
      mask prompts: N "Numerator:"; D "Denominator:"; Y0 "Initial output:"; U0 "Initial input:"
      mask help: Vector expressions for numerator, and denominator. Coefficients are in descending powers of s.
      mask init:
      | [A,B,C,Dd]=tf2ss(N,D);if (isempty(Y0));[m,n]=size(A);X0=zeros(1,m); end; if (isempty(U0));[m,p]=size(B);U0=zeros(1,p);end;X0=getxo(A,B,C,Dd,U0,Y0,0);
      mask Help: Specify the initial output for the transfer function.  An optimization routine attempts to determine the appropriate initial states so that the specified initial output is achieved.  For more details, see the m-file getxo.m
      mask Display: dpoly(N,D,'s')
  real : Subsystem  mask(Transfer Function with Initial Outputs){N=[1], D=[to 1], Y0=0, U0=0}
      mask prompts: N "Numerator:"; D "Denominator:"; Y0 "Initial output:"; U0 "Initial input:"
      mask help: Vector expressions for numerator, and denominator. Coefficients are in descending powers of s.
      mask init:
      | [A,B,C,Dd]=tf2ss(N,D);if (isempty(Y0));[m,n]=size(A);X0=zeros(1,m); end; if (isempty(U0));[m,p]=size(B);U0=zeros(1,p);end;X0=getxo(A,B,C,Dd,U0,Y0,0);
      mask Help: Specify the initial output for the transfer function.  An optimization routine attempts to determine the appropriate initial states so that the specified initial output is achieved.  For more details, see the m-file getxo.m
      mask Display: dpoly(N,D,'s')
  Out : Outport  VectorParamsAs1DForOutWhenUnconnected=off
  wires:
  Complex to Real-Imag/1 -> real/1(In1)
  Complex to Real-Imag/2 -> imag/1(In1)
  In/1 -> Complex to Real-Imag/1
  Real-Imag to Complex/1 -> Out/1
  real/1(Out1) -> Real-Imag to Complex/1
  imag/1(Out1) -> Real-Imag to Complex/2

== system ZEH_PV_grid/L1/Break Alg. Loop 1/imag ==
  In1 : Inport
  State Space : StateSpace  A=A  B=B  C=C  D=Dd  InitialCondition=X0
  Out1 : Outport  InitialOutput=0  VectorParamsAs1DForOutWhenUnconnected=off
  wires:
  State Space/1 -> Out1/1
  In1/1 -> State Space/1

== system ZEH_PV_grid/L1/Break Alg. Loop 1/real ==
  In1 : Inport
  State Space : StateSpace  A=A  B=B  C=C  D=Dd  InitialCondition=X0
  Out1 : Outport  InitialOutput=0  VectorParamsAs1DForOutWhenUnconnected=off
  wires:
  State Space/1 -> Out1/1
  In1/1 -> State Space/1

== system ZEH_PV_grid/L10/Break Alg. Loop 1/imag ==
  In1 : Inport
  State Space : StateSpace  A=A  B=B  C=C  D=Dd  InitialCondition=X0
  Out1 : Outport  InitialOutput=0  VectorParamsAs1DForOutWhenUnconnected=off
  wires:
  In1/1 -> State Space/1
  State Space/1 -> Out1/1

== system ZEH_PV_grid/L10/Break Alg. Loop 1/real ==
  In1 : Inport
  State Space : StateSpace  A=A  B=B  C=C  D=Dd  InitialCondition=X0
  Out1 : Outport  InitialOutput=0  VectorParamsAs1DForOutWhenUnconnected=off
  wires:
  In1/1 -> State Space/1
  State Space/1 -> Out1/1

== system ZEH_PV_grid/L11/Break Alg. Loop 1/imag ==
  In1 : Inport
  State Space : StateSpace  A=A  B=B  C=C  D=Dd  InitialCondition=X0
  Out1 : Outport  InitialOutput=0  VectorParamsAs1DForOutWhenUnconnected=off
  wires:
  State Space/1 -> Out1/1
  In1/1 -> State Space/1

== system ZEH_PV_grid/L11/Break Alg. Loop 1/real ==
  In1 : Inport
  State Space : StateSpace  A=A  B=B  C=C  D=Dd  InitialCondition=X0
  Out1 : Outport  InitialOutput=0  VectorParamsAs1DForOutWhenUnconnected=off
  wires:
  State Space/1 -> Out1/1
  In1/1 -> State Space/1

== system ZEH_PV_grid/L2/Break Alg. Loop 1/imag ==
  In1 : Inport
  State Space : StateSpace  A=A  B=B  C=C  D=Dd  InitialCondition=X0
  Out1 : Outport  InitialOutput=0  VectorParamsAs1DForOutWhenUnconnected=off
  wires:
  In1/1 -> State Space/1
  State Space/1 -> Out1/1
